simulink model "a_model"  (R2023a)
settings: Solver=VariableStepAuto  StartTime=0.0  StopTime=10  RelTol=1e-3
undefined symbols (not defined in the file or in its folder): DiscIntNeverNeededParam
settings Model: Creator=under  LastModifiedBy=under

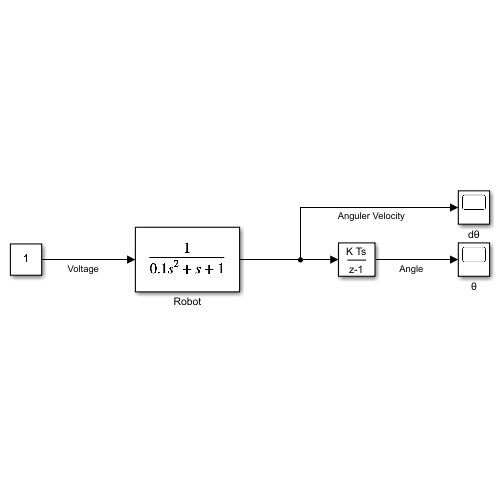
[thumbnail: Simulink's stored preview of the top-level diagram]
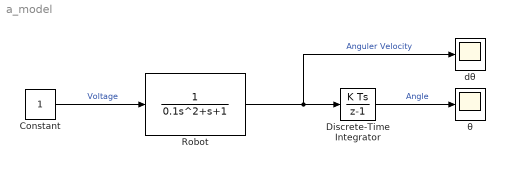
== system a_model ==
  Constant : Constant
  Discrete-Time Integrator : DiscreteIntegrator  SampleTime=1e-3  ICPrevOutput=DiscIntNeverNeededParam  ICPrevScaledInput=DiscIntNeverNeededParam
  Robot : TransferFcn  Denominator=[0.1 1 1]
  dθ : Scope
  θ : Scope
  wires:
  Constant/1 -> Robot/1  "Voltage"
  Robot/1 -> Discrete-Time Integrator/1, dθ/1  "Anguler Velocity"
  Discrete-Time Integrator/1 -> θ/1  "Angle"
